simulink model "base_1fm"  (R2016b)
settings: Solver=VariableStepAuto  StartTime=0.0  StopTime=10.0  RelTol=1e-3
values from neighbouring files (symbols this model uses):
  Lb = 0.07    [base_1fm_parameters.m]
  Lf = 0.238    [base_1fm_parameters.m]
  Lu = 0.153    [base_1fm_parameters.m]
  sampleTime = 0.001    [base_1fm_parameters.m]
undefined symbols (not defined in the file or in its folder): DiscIntNeverNeededParam, RobotStruct
undefined symbols (not defined in the file): RobotStruct_FM1
libraries: simulink x27, VariousBlocksLibrary x4, FMLibrary_v2 x2, UsefulBlocksLibrary x2, simulink_extras x2, FM_Library x1
(part 3 of 3)

== matlab function base_1fm/Robot1/DataFromEtherCAT/FromActuator2/CalculateJointVelocity/FOAW ==
  data: x input; xdot output; sampleTime parameter; noise input
function xdot = foaw(x, sampleTime, noise)
%#codegen

SIZE = 100; % number of samples in buffer
NOISE = noise;
Ts = sampleTime;

persistent posbuffer;
persistent buffercntr;

% initialize buffer
if isempty(posbuffer)
    posbuffer = zeros(SIZE,1); % 1D case for now
    buffercntr = 0;
end

% fill buffer: shift data and add new value (loose oldest sample)
posbuffer = [posbuffer(2:end); x];
buffercntr = buffercntr + 1;
if buffercntr > SIZE, buffercntr = SIZE; end;

% if buffercntr = 1, only 1 data point is available, and you can't make a
% velocity prediction based on 1 data point. Set velocity ot 0, and return
% function
xdot = 0;
if buffercntr <= 3
    return;
end

for n = 1:buffercntr-1 % n = window size
        
    % step 2
    currentpos = posbuffer(end);

    % step 3 - calculate LS approximation of slope (hence velocity)
    b = n*sum(posbuffer(end-n:end)) - 2*sum(posbuffer(end-n:end).*(n:-1:0)');
    b = b / (Ts*n*(n+1)*(n+2)/6);

    % step 4 - check whether the line an + bn*Ts passes through all points inside the 
    % window within the uncertainty band of each point 
    jj = 0:n;
    yk_hat = currentpos-(b*jj*Ts);
    yk = posbuffer(end-jj)';
    if any(abs(yk_hat-yk) > NOISE)
        break;
    end

    xdot = b;
end

== matlab function base_1fm/Robot1/DataFromEtherCAT/FromActuator1/CalculateJointVelocity/FOAW ==
  data: x input; xdot output; sampleTime parameter; noise input
function xdot = foaw(x, sampleTime, noise)
%#codegen

SIZE = 100; % number of samples in buffer
NOISE = noise;
Ts = sampleTime;

persistent posbuffer;
persistent buffercntr;

% initialize buffer
if isempty(posbuffer)
    posbuffer = zeros(SIZE,1); % 1D case for now
    buffercntr = 0;
end

% fill buffer: shift data and add new value (loose oldest sample)
posbuffer = [posbuffer(2:end); x];
buffercntr = buffercntr + 1;
if buffercntr > SIZE, buffercntr = SIZE; end;

% if buffercntr = 1, only 1 data point is available, and you can't make a
% velocity prediction based on 1 data point. Set velocity ot 0, and return
% function
xdot = 0;
if buffercntr <= 3
    return;
end

for n = 1:buffercntr-1 % n = window size
        
    % step 2
    currentpos = posbuffer(end);

    % step 3 - calculate LS approximation of slope (hence velocity)
    b = n*sum(posbuffer(end-n:end)) - 2*sum(posbuffer(end-n:end).*(n:-1:0)');
    b = b / (Ts*n*(n+1)*(n+2)/6);

    % step 4 - check whether the line an + bn*Ts passes through all points inside the 
    % window within the uncertainty band of each point 
    jj = 0:n;
    yk_hat = currentpos-(b*jj*Ts);
    yk = posbuffer(end-jj)';
    if any(abs(yk_hat-yk) > NOISE)
        break;
    end

    xdot = b;
end

== matlab function base_1fm/Robot1/DataToEtherCAT/FTSensorError/MATLAB Function ==
  data: ForcesTorques input; e output; MaxForcesTorques input
function e = fcn(ForcesTorques, MaxForcesTorques)

% throw error when any of the forces/torques go over a max allowable value
if any(abs(ForcesTorques) > MaxForcesTorques) 
    e = 1;
else
    e = 0;
end

== matlab function base_1fm/Robot1/DataFromEtherCAT/FromActuator2/CalibrateAbsEncoder ==
  data: encoderPosition input; JointPosition_AbsEnc_rad output; offset input
function JointPosition_AbsEnc_rad = CalibrateAbsoluteEncoder(encoderPosition, offset)
%#codegen

% unwrap encoder angle (in case the encoder goes through 0
encoderPosition = unwrap(encoderPosition);

% remove offset
JointPosition_AbsEnc_rad = encoderPosition - offset;

% since the absolute encoder is mounted upside-down, negate the
% jointposition angle
JointPosition_AbsEnc_rad = -JointPosition_AbsEnc_rad;

== matlab function base_1fm/Robot1/DataFromEtherCAT/FromActuator2/CalibrateMotorPosition     ==
  data: JointPosition_IncEnc_rad output; MotorPosition_rad input; MotorPositionCalibrated_rad output; transmissionRatio parameter; JointPosition_AbsEnc_rad input; Calibrate input
function [JointPosition_IncEnc_rad,MotorPositionCalibrated_rad]...
    = CalibrateMotorPosition( MotorPosition_rad, transmissionRatio, JointPosition_AbsEnc_rad, Calibrate)
%#codegen

% This block includes calibration such that (ideally) the motor angle is
% zero when the joint angle and spring deflection are zero as well. Before
% the calibration has occurred, the output of this function is -1e9*. This
% is chosen such that the value is always outside the allowed motor angle
% range; this prevents the drive from being allowed to turn on.
% 
% * I wanted to use -inf as starting function, but I'm not sure whether
%   that will be handled correctly in all cases.

persistent isCalibrated;
persistent offset;

if isempty(isCalibrated) % no calibration needed
    isCalibrated = 1;
    offset = 0;
end;


if Calibrate
%     if ~isempty(JointPosition_AbsEnc_rad)
        target_pos_mot_rad = transmissionRatio * JointPosition_AbsEnc_rad; % This is what we should read
%         target_pos_mot_rad = CalibrationAngle; % This is what we should read / fix for now
        offset = target_pos_mot_rad - MotorPosition_rad; % calculate offset
%     else
%         % no absolute encoder data available, offset is zero
%         offset = 0;
%     end
    isCalibrated = 1;
end;

% if already calibrated, calculate calibrated motor angle
if isCalibrated
    MotorPositionCalibrated_rad = MotorPosition_rad + offset;
    JointPosition_IncEnc_rad = MotorPositionCalibrated_rad / transmissionRatio;
else
    MotorPositionCalibrated_rad = MotorPosition_rad;
    JointPosition_IncEnc_rad = MotorPositionCalibrated_rad / transmissionRatio;
end;

== matlab function base_1fm/Robot1/DataFromEtherCAT/FromActuator2/CheckOperationEnabled ==
  data: u input; y output
function y = fcn(u)
%#codegen

mask  = bin2dec('0000000001101111');
match = bin2dec('0000000000100111');

masked = bitand(u,mask);
if masked==match
    y=1;
else
    y=0;
end;

== matlab function base_1fm/Robot1/Controller/PD + Nonlinear ID/AFFC/AFFC ==
  data: p output; t input; q input; qdot input; qddot input; e input; tau output; Lf parameter; Lu parameter; Lb parameter; w input
function [p,tau] = fcn(t, q, qdot, qddot, e, Lf, Lu, Lb,w)

persistent p_;

if isempty(p_)
%     p_ = [0.00173;0.00159;0.048;0.07889;-0.00389;0.08784;-0.00474];
    p_ = zeros(7,1);
end


% jacobians
J = func_eq_Je(q(1),q(2),Lf,Lu,Lb);
Jdot = func_eq_Jedot(q(1),q(2),qdot(1),qdot(2),Lf,Lu,Lb);

% create Psi
Psi = [diag([qddot(1) qddot(2)]) J'*J*qddot+J'*Jdot*qdot [sign(qdot(1)) qdot(1); 0 0] [0 0;sign(qdot(2)) qdot(2)] ];

% learning matrix Gamma
eta = 0.95*exp(-t/150) + 0.05;
% eta = 1;
% wI = 1e-3;
% wme = 5e-2;
% wfd = 1e-3;
% wfs = 1e-3;

wI = w(1);
wme = w(2);
wfd = w(3);
wfs = w(4);

Gamma = eta*diag([wI wI wme wfs wfd wfs wfd]);

% update p (parameter vector)
% learning rule
dp = Gamma*Psi'*e;
p_ = p_ + dp;

% Psi = [diag([qddot(1) qddot(2)]) J'*J*qddot+J'*Jdot*qdot [ssign(qdot(1)) qdot(1); 0 0] [0 0;ssign(qdot(2)) qdot(2)] ];

% feedforward torque
tau = Psi*p_;

p = p_;

function y = ssign(u,beta)
% soft sign
if nargin == 1
    beta = 150;
end

y = 2./(1+exp(-beta*u))-1;

== stateflow chart base_1fm/Robot1/StateMachineLocal/SystemLocalStateMachine ==
  settings: initializeOutput=1
  state Operational
    state Calibration
      en:
      systemState = 2;
      velBelowThreshold = false;
      du:
      velBelowThreshold = checkVelThreshold(0.001 );
      state JointVelLarge
      state JointVelSmall
      state DoCalibration
        en: systemState = 201;
      state CalibrationDone
        en: systemState = 299;
      (default) -> JointVelLarge
      JointVelSmall -> JointVelLarge [order 1] : [!velBelowThreshold]
      JointVelLarge -> JointVelSmall : [velBelowThreshold]
      JointVelSmall -> DoCalibration [order 2] : after(2,sec)
      DoCalibration -> CalibrationDone
    state Homing
      en:
      systemState = reqSystemState;
      isAtHome = false;
      du:
      isAtHome = checkEndpointPosition(homeLocationSize);
      state NotAtHome
      state AtHome
      state HomingDone
        en: systemState = 399;
      (default) -> NotAtHome
      AtHome -> NotAtHome [order 1] : [!isAtHome]
      NotAtHome -> AtHome : [isAtHome]
      AtHome -> HomingDone [order 2] : after(1,sec)
    state Run
      en: systemState = 4;
    (default) -> Calibration
    CalibrationDone -> Homing : [reqSystemState == 301 || reqSystemState == 302]
    Run -> Homing : [reqSystemState==3]
    HomingDone -> Run : [reqSystemState==4]
  state Idle
    en:
    systemState = 0;
  state Init
    en:
    systemState = 1;
    du:
    isInitialized = true;
  state Error
    en: systemState=-1;
  (default) -> Idle
  Init -> Operational [order 1] : [isInitialized]
  Idle -> Init [order 2] : [reqSystemState==1]
  Init -> Idle [order 3] : [reqSystemState==0]
  Error -> Idle : [!error   && reqSystemState==0]
  Init -> Error [order 2] : [error]
  Idle -> Error [order 1] : [error]
  Operational -> Idle [order 2] : [reqSystemState==0]
  Operational -> Error [order 1] : [error]
  data: threshold function_input double; velIsUnderThreshold function_output boolean; threshold function_input double; isAtEndpoint function_output boolean; reqSystemState input double; currentSystemState output double; error input boolean; x input double; xdot input double; HomePosition input double; isAtHome local boolean; velBelowThreshold local boolean; isInitialized local double; homeLocationSize input
  function velIsUnderThreshold = checkVelThreshold(threshold):
    | function velIsUnderThreshold = checkVelThreshold(threshold)
    |  
    | velIsUnderThreshold = all(abs(xdot) <= threshold);
  function isAtEndpoint = checkEndpointPosition(threshold):
    | function isAtEndpoint = checkEndpointPosition(threshold)
    | % check whether the endpoint position is within a specified circle with
    | % radius threshold and midopoint HomePosition
    | 
    | % calculate distance between home position and joint positions
    | d = sqrt(sum((HomePosition - x).^2));
    | 
    | if imag(d) || isinf(d) || isnan(d)
    |     isAtEndpoint = false;
    | else
    |     isAtEndpoint = d <= threshold;
    | end

== matlab function base_1fm/Robot1/StateMachineLocal/Encode system state change ==
  data: stateChanged input; state input; systemStateChanged output
function systemStateChanged  = fcn(stateChanged,state)

systemStateChanged = 0;


if stateChanged
    switch(state)
        case 201 % do calibration
            systemStateChanged = 1;
    end
end

== matlab function base_1fm/Robot1/DataFromEtherCAT/Calculate Arrange Joint and Op Space/forward kinematics/forward kinematics ==
  data: q input; x output size=[2 1]; Lf parameter; Lu parameter; Lb parameter
function x = FK(q, Lf, Lu, Lb)
%#codegen

% Calculate the endpoint position (forward kinematics)
% Note that the function func_eq_FK needs to be in the libraries/kinematis_functions folder


x = func_eq_FK(q(1),q(2),Lf,Lu,Lb);

== matlab function base_1fm/Robot1/DataFromEtherCAT/FromActuator2/DecodeActualTorque ==
  data: JointTorque_Act_Nm output; MotorCurrent_Act_IU input int16; transmissionRatio parameter; drivePeakCurrent parameter; motorTorqueConstant parameter
function JointTorque_Act_Nm = DecodeActualTorque(MotorCurrent_Act_IU, transmissionRatio, drivePeakCurrent, motorTorqueConstant)
%#codegen
%

% convert incremental units to motor torque value. See the technosoft CoE
% manual for the decoding
torquemotor_act = motorTorqueConstant * (double(MotorCurrent_Act_IU)*2*drivePeakCurrent / 65520);

% motor torque to joint torque (transmission). Negate due to sign change
% due to transmission.
JointTorque_Act_Nm = torquemotor_act * transmissionRatio;

== matlab function base_1fm/Robot1/DataFromEtherCAT/FromActuator2/DecodeEncoder_AbsEnc ==
  data: Encoder_counts input; EncoderCounts_rev parameter; EncoderPosition_rad output
function EncoderPosition_rad = ...
    DecodeEncoder(Encoder_counts, EncoderCounts_rev)
%#codegen

% This block decodes the motor encoder counts to the motor angle

EncoderPosition_rad = (double(Encoder_counts) / EncoderCounts_rev * 2 * pi);

== matlab function base_1fm/Robot1/Controller/inverse kinematics1 ==
  data: x input; q output size=[2 1]; Lf parameter; Lu parameter; Lb parameter
function q  = IK(x,Lf,Lu,Lb)
%#codegen

% inverse dynamics
q = func_eq_IK(x(1),x(2),Lf,Lu,Lb);

== matlab function base_1fm/Robot1/DataFromEtherCAT/FromActuator2/DecodeEncoder_IncEnc ==
  data: Encoder_counts input; EncoderCounts_rev parameter; EncoderPosition_rad output
function EncoderPosition_rad = ...
    DecodeEncoder(Encoder_counts, EncoderCounts_rev)
%#codegen

% This block decodes the motor encoder counts to the motor angle

EncoderPosition_rad = (double(Encoder_counts) / EncoderCounts_rev * 2 * pi);

== matlab function base_1fm/Robot1/DataFromEtherCAT/FromActuator1/CalibrateMotorPosition     ==
  data: JointPosition_IncEnc_rad output; MotorPosition_rad input; MotorPositionCalibrated_rad output; transmissionRatio parameter; JointPosition_AbsEnc_rad input; Calibrate input
function [JointPosition_IncEnc_rad,MotorPositionCalibrated_rad]...
    = CalibrateMotorPosition( MotorPosition_rad, transmissionRatio, JointPosition_AbsEnc_rad, Calibrate)
%#codegen

% This block includes calibration such that (ideally) the motor angle is
% zero when the joint angle and spring deflection are zero as well. Before
% the calibration has occurred, the output of this function is -1e9*. This
% is chosen such that the value is always outside the allowed motor angle
% range; this prevents the drive from being allowed to turn on.
% 
% * I wanted to use -inf as starting function, but I'm not sure whether
%   that will be handled correctly in all cases.

persistent isCalibrated;
persistent offset;

if isempty(isCalibrated) % no calibration needed
    isCalibrated = 1;
    offset = 0;
end;


if Calibrate
%     if ~isempty(JointPosition_AbsEnc_rad)
        target_pos_mot_rad = transmissionRatio * JointPosition_AbsEnc_rad; % This is what we should read
%         target_pos_mot_rad = CalibrationAngle; % This is what we should read / fix for now
        offset = target_pos_mot_rad - MotorPosition_rad; % calculate offset
%     else
%         % no absolute encoder data available, offset is zero
%         offset = 0;
%     end
    isCalibrated = 1;
end;

% if already calibrated, calculate calibrated motor angle
if isCalibrated
    MotorPositionCalibrated_rad = MotorPosition_rad + offset;
    JointPosition_IncEnc_rad = MotorPositionCalibrated_rad / transmissionRatio;
else
    MotorPositionCalibrated_rad = MotorPosition_rad;
    JointPosition_IncEnc_rad = MotorPositionCalibrated_rad / transmissionRatio;
end;

== matlab function base_1fm/Robot1/Controller/homing - active/Filter1 ==
  data: x input; OmegaFilter input; y output; sampleTime parameter
function y = Filter2ndOrder(x, OmegaFilter, sampleTime)
%#codegen

persistent yd_prev y_prev;
if isempty(yd_prev)
    yd_prev = 0; 
    y_prev = 0; %Derivative of the above signal
end;

% Do 2nd order filtering with given omega and zeta=0.7; input of filter
% is vel_inc_sampleTime_unfilt; output is y (we assign to vel_inc_s
% later). 
if OmegaFilter==0 || isinf(OmegaFilter)
    y=x;
    y_prev=y;
    yd_prev =0;
else
    zeta = 0.7;
    ydd = OmegaFilter^2 * (x - y_prev) - 2*zeta*OmegaFilter* yd_prev;
    yd = yd_prev + ydd * sampleTime;
    y = y_prev + yd * sampleTime;

    y_prev = y; yd_prev = yd;
end;

== matlab function base_1fm/Haptics/Hypotrochoid trajectory for AFFC/hypotrochoidal trajectory ==
  data: t input; p output; v output; a output; T input; n input; hstart input; hend input; wstart input; wend input
function [p,v,a] = fcn(t,T,n,hstart,hend,wstart,wend)
%#codegen

p = func_p_hypothrochoid(t,T,n,hstart,hend,wstart,wend);
v = func_v_hypothrochoid(t,T,n,hstart,hend,wstart,wend);
a = func_a_hypothrochoid(t,T,n,hstart,hend,wstart,wend);

== matlab function base_1fm/Robot1/DataToEtherCAT/ToActuator1/DriveEnableLogic/64_DriveError/CountHowLongEnableWasTrue ==
  data: u input; y output
function y = fcn(u)
%#codegen
%
% This block counts how many samples the input has been on (true). As soon
% as the input goes false, the counter is reset.
persistent onCounter;

if isempty(onCounter)
    onCounter = 0;
end;

if u == 1
    onCounter = onCounter + 1;
else
    % u == 0
    onCounter = 0;
end;
y = onCounter;

== matlab function base_1fm/Robot1/DataFromEtherCAT/Calculate Arrange Joint and Op Space/forward kinematics/Je ==
  data: q input; Je output size=[2 2]; Lf parameter; Lu parameter; Lb parameter
function Je = Je( q, Lf, Lu, Lb)
%#codegen

% Calculate the Jacobian for this particular device configuration.
% Note that the function func_eq_Je needs to be in the libraries/kinematis_functions folder

% jacobians
Je = func_eq_Je(q(1),q(2),Lf,Lu,Lb);

== matlab function base_1fm/Robot1/DataFromEtherCAT/Calculate Arrange Joint and Op Space/forward kinematics/Jedot ==
  data: q input; qdot input; Jedot output size=[2 2]; Lf parameter; Lu parameter; Lb parameter
function Jedot = Jedot( q, qdot, Lf, Lu, Lb)
%#codegen

% Calculate the time derivative of the Jacobian for this particular device configuration.
% Note that the function func_eq_Je needs to be in the libraries/kinematis_functions folder


% jacobians
Jedot = func_eq_Jedot(q(1),q(2),qdot(1),qdot(2),Lf,Lu,Lb);

== matlab function base_1fm/Robot1/DataFromEtherCAT/FTSensor_K6D27/CorrectOffset ==
  data: u_in input; u_out output; reset input; corrected output
function [u_out,corrected] = CorrectOffset(u_in,reset)
%#codegen

persistent data_ offset_ counter_ corrected_;
N = 1000;

% initialize
if isempty(data_)
    data_ = zeros(size(u_in,1), N);
    offset_ = zeros(size(u_in));
    counter_ = 1;
    corrected_ = 0;
end

if (counter_ <= N)
    data_(:,counter_) = u_in;
end

counter_ = counter_ + 1;
if reset
    counter_ = 1;
end

% calculate mean
if counter_ == N
    corrected_ = 1;
    offset_ = mean(data_,2);
end

corrected = corrected_;
u_out = u_in - offset_;

== matlab function base_1fm/Robot1/DataFromEtherCAT/FromActuator1/CheckOperationEnabled ==
  data: u input; y output
function y = fcn(u)
%#codegen

mask  = bin2dec('0000000001101111');
match = bin2dec('0000000000100111');

masked = bitand(u,mask);
if masked==match
    y=1;
else
    y=0;
end;

== matlab function base_1fm/Robot1/DataFromEtherCAT/Calculate Arrange Joint and Op Space/IK all joints ==
  data: x input; q_all output; Lf parameter; Lu parameter; Lb parameter
function q_all = IK_all(x,Lf,Lu,Lb)
%#codegen

if (x(2) >= 0.07)
    q_all = func_eqs_IK_all(x(1),x(2),Lf,Lu,Lb);
else
    x = [0;0.07];
    q_all = func_eqs_IK_all(x(1),x(2),Lf,Lu,Lb);
end

== matlab function base_1fm/Robot1/DataFromEtherCAT/Calculate Arrange Joint and Op Space/forward kinematics/calculate xddot ==
  data: qddot input; qdot input size=[2 1]; J input; xddot output size=[2 1]; Jdot input
function xddot = calc_xddot(qddot, qdot, J, Jdot)
%#codegen

xddot = J*qddot + Jdot*qdot;

== matlab function base_1fm/Robot1/Controller/inverse kinematics ==
  data: x input; xdot input; xddot input; q output size=[2 1]; Lf parameter; Lu parameter; Lb parameter; qdot output; qddot output
function [q,qdot,qddot] = IK(x,xdot,xddot,Lf,Lu,Lb)
%#codegen

% inverse dynamics
q = func_eq_IK(x(1),x(2),Lf,Lu,Lb);

% jacobians
Je = func_eq_Je(q(1),q(2),Lf,Lu,Lb);

% calculate qdot
qdot = pinv(Je)*xdot;

% calculate qddot
Jedot = func_eq_Jedot(q(1),q(2),qdot(1),qdot(2),Lf,Lu,Lb);
qddot = pinv(Je)*(xddot-Jedot*qdot);

== matlab function base_1fm/Robot1/DataToEtherCAT/ToActuator1/DriveEnableLogic/CreateSingleErrorValue/MATLAB Function ==
  data: errors input; out output
function out = errorToPowerOf2(errors)
%#codegen

% if size(errors,1) > size(errors,2)
%     errors = errors.';
% end
out = sum(errors.*(2.^(0:(length(errors)-1)).'));

== matlab function base_1fm/Robot1/DataToEtherCAT/ToActuator1/DriveEnableLogic/enableDrive (CoE) ==
  data: ControlWord output; enable input; TimePerState_ms input
function ControlWord = enabledrive(enable, TimePerState_ms)
%#codegen
%
% Input arguments:
% enable:
%   0: Disable drive
%   Any non-zero: enable drive.
% TimePerState_ms:
%   A four-element array containing the time in ms for each state (states
%   are: 0, 128, 6, 7. The final state, 15, is kept until drive needs to be
%   disabled again.
%
% Changing enable forces the initialize-sequence to run
persistent previousEnable;
persistent counter;
if isempty(previousEnable)
    previousEnable = enable; % No enabling of the drive at startup
    counter = 1e6;
end;

if enable~=previousEnable
    counter = 0;
end;
previousEnable = enable;

TimePerState_cum = cumsum(TimePerState_ms);

if enable~=0
    counter = counter+1;
    if counter < TimePerState_cum(1);
        ControlWord_ = 0;
    elseif counter < TimePerState_cum(2);
        ControlWord_ = 128;
    elseif counter < TimePerState_cum(3);
        ControlWord_ = 6;
    elseif counter < TimePerState_cum(4);
        ControlWord_ = 7;
    else
        ControlWord_ = 15;
    end
else
    ControlWord_ = 6;
end

ControlWord = uint16(ControlWord_);

== matlab function base_1fm/Robot1/DataToEtherCAT/ToActuator1/EncodeDesiredTorque ==
  data: MotorTorque_Des_IU output int16; JointTorque_Des_Nm input; transmissionRatio parameter; motorTorqueConstant parameter; drivePeakCurrent parameter
function MotorTorque_Des_IU = EncodeDesiredTorque(JointTorque_Des_Nm, transmissionRatio, motorTorqueConstant, drivePeakCurrent)
%#codegen
% Calculate the target torque in incremental units for a desired joint
% torque.

% compute torque at motor (negate because sign change due to transmission)
torque_motor = JointTorque_Des_Nm / transmissionRatio; 

% desired current (i_des) = torque_motor / kt (torque constant)
i_des = torque_motor / motorTorqueConstant;

% calculate the target torque in incremental units [IU], see CoE manual
% Technosoftmotion
MotorTorque_Des_IU = int16( 65520*i_des / (2*drivePeakCurrent) );

== matlab function base_1fm/Robot1/DataToEtherCAT/ToActuator/DriveEnableLogic/64_DriveError/CountHowLongEnableWasTrue ==
  data: u input; y output
function y = fcn(u)
%#codegen
%
% This block counts how many samples the input has been on (true). As soon
% as the input goes false, the counter is reset.
persistent onCounter;

if isempty(onCounter)
    onCounter = 0;
end;

if u == 1
    onCounter = onCounter + 1;
else
    % u == 0
    onCounter = 0;
end;
y = onCounter;

== matlab function base_1fm/Robot1/DataFromEtherCAT/FromActuator1/DecodeActualTorque ==
  data: JointTorque_Act_Nm output; MotorCurrent_Act_IU input int16; transmissionRatio parameter; drivePeakCurrent parameter; motorTorqueConstant parameter
function JointTorque_Act_Nm = DecodeActualTorque(MotorCurrent_Act_IU, transmissionRatio, drivePeakCurrent, motorTorqueConstant)
%#codegen
%

% convert incremental units to motor torque value. See the technosoft CoE
% manual for the decoding
torquemotor_act = motorTorqueConstant * (double(MotorCurrent_Act_IU)*2*drivePeakCurrent / 65520);

% motor torque to joint torque (transmission). Negate due to sign change
% due to transmission.
JointTorque_Act_Nm = torquemotor_act * transmissionRatio;

== matlab function base_1fm/Robot1/DataFromEtherCAT/FromActuator1/DecodeEncoder_AbsEnc ==
  data: Encoder_counts input; EncoderCounts_rev parameter; EncoderPosition_rad output
function EncoderPosition_rad = ...
    DecodeEncoder(Encoder_counts, EncoderCounts_rev)
%#codegen

% This block decodes the motor encoder counts to the motor angle

EncoderPosition_rad = (double(Encoder_counts) / EncoderCounts_rev * 2 * pi);

== matlab function base_1fm/Robot1/DataFromEtherCAT/FromActuator1/DecodeEncoder_IncEnc ==
  data: Encoder_counts input; EncoderCounts_rev parameter; EncoderPosition_rad output
function EncoderPosition_rad = ...
    DecodeEncoder(Encoder_counts, EncoderCounts_rev)
%#codegen

% This block decodes the motor encoder counts to the motor angle

EncoderPosition_rad = (double(Encoder_counts) / EncoderCounts_rev * 2 * pi);

== matlab function base_1fm/Robot1/DataFromEtherCAT/FromActuator1/CalibrateAbsEncoder ==
  data: encoderPosition input; JointPosition_AbsEnc_rad output; offset input
function JointPosition_AbsEnc_rad = CalibrateAbsoluteEncoder(encoderPosition, offset)
%#codegen

% unwrap encoder angle (in case the encoder goes through 0
encoderPosition = unwrap(encoderPosition);

% remove offset
JointPosition_AbsEnc_rad = encoderPosition - offset;

% since the absolute encoder is mounted upside-down, negate the
% jointposition angle
JointPosition_AbsEnc_rad = -JointPosition_AbsEnc_rad;

== matlab function base_1fm/Robot1/DataToEtherCAT/ToActuator/DriveEnableLogic/CreateSingleErrorValue/MATLAB Function ==
  data: errors input; out output
function out = errorToPowerOf2(errors)
%#codegen

% if size(errors,1) > size(errors,2)
%     errors = errors.';
% end
out = sum(errors.*(2.^(0:(length(errors)-1)).'));

== matlab function base_1fm/Robot1/DataToEtherCAT/ToActuator/DriveEnableLogic/enableDrive (CoE) ==
  data: ControlWord output; enable input; TimePerState_ms input
function ControlWord = enabledrive(enable, TimePerState_ms)
%#codegen
%
% Input arguments:
% enable:
%   0: Disable drive
%   Any non-zero: enable drive.
% TimePerState_ms:
%   A four-element array containing the time in ms for each state (states
%   are: 0, 128, 6, 7. The final state, 15, is kept until drive needs to be
%   disabled again.
%
% Changing enable forces the initialize-sequence to run
persistent previousEnable;
persistent counter;
if isempty(previousEnable)
    previousEnable = enable; % No enabling of the drive at startup
    counter = 1e6;
end;

if enable~=previousEnable
    counter = 0;
end;
previousEnable = enable;

TimePerState_cum = cumsum(TimePerState_ms);

if enable~=0
    counter = counter+1;
    if counter < TimePerState_cum(1);
        ControlWord_ = 0;
    elseif counter < TimePerState_cum(2);
        ControlWord_ = 128;
    elseif counter < TimePerState_cum(3);
        ControlWord_ = 6;
    elseif counter < TimePerState_cum(4);
        ControlWord_ = 7;
    else
        ControlWord_ = 15;
    end
else
    ControlWord_ = 6;
end

ControlWord = uint16(ControlWord_);

== matlab function base_1fm/Robot1/DataToEtherCAT/ToActuator/EncodeDesiredTorque ==
  data: MotorTorque_Des_IU output int16; JointTorque_Des_Nm input; transmissionRatio parameter; motorTorqueConstant parameter; drivePeakCurrent parameter
function MotorTorque_Des_IU = EncodeDesiredTorque(JointTorque_Des_Nm, transmissionRatio, motorTorqueConstant, drivePeakCurrent)
%#codegen
% Calculate the target torque in incremental units for a desired joint
% torque.

% compute torque at motor (negate because sign change due to transmission)
torque_motor = JointTorque_Des_Nm / transmissionRatio; 

% desired current (i_des) = torque_motor / kt (torque constant)
i_des = torque_motor / motorTorqueConstant;

% calculate the target torque in incremental units [IU], see CoE manual
% Technosoftmotion
MotorTorque_Des_IU = int16( 65520*i_des / (2*drivePeakCurrent) );

== matlab function base_1fm/Robot1/DataFromEtherCAT/FTSensor_K6D27/SensorOutputToForce1 ==
  data: FT output; u input; calibrationMatrix input; offset input
function FT = VtoF(u, calibrationMatrix, offset)
%#codegen

% ME supplies a zero offset voltages. If 
if ~isempty(offset)
    u = u + offset;
end

% Calculate forces and torques (in sensor space)
FT = calibrationMatrix*u;

== matlab function base_1fm/Robot1/DataFromEtherCAT/FTSensor_K6D27/SensorToOperationalSpace ==
  data: q_all input; Fs input; FTOpSpace output
function FTOpSpace = ForceSensorToOperationalSpace(q_all,Fs)
%#codegen

% select correct angles. Note! During assembly we weren't very consistent
% to which forearm the sensor is fixed. For FM1 (green), the sensor is
% attached to arm 2, hence the rotation matrics are made using angles
% theta1 and theta2
% rotation matrices (I derived them from actuator 1 to endpoint, but
% transformation is other way around (i.e. inverse). Since inverse calculation 
% could take some time, Could be done by
% negating the angles instead of inverse of matrix.
q1 = q_all(1);
q2 = (pi-q_all(2)); % pi-theta2 since theta2 is the internal angle of this joint

R = [-cos(q1+q2) sin(q1+q2);-sin(q1+q2) -cos(q1+q2)];

% transform force
FTOpSpace = R*Fs(1:2);

== matlab function base_1fm/Robot1/DataToEtherCAT/WorkspacePositionGuard/CheckForSingularity ==
  data: J input; kappa output
function kappa = conditionnumber(J)
%#codegen

kappa = norm(pinv(J))*norm(J);

== matlab function base_1fm/Robot1/DataToEtherCAT/WorkspacePositionGuard/CheckInternalAngles ==
  data: theta input; angleError output; isCalibrated input
function angleError = checkInternalErrors(theta,isCalibrated)
%#codegen

angleError = 0;

if isCalibrated
    % check whether theta2 or theta4 are smaller than 0.95*pi. If larger, throw
    % error
    if any(theta([2 4]) >= 0.95*pi)
        angleError = 1;
    end
end

== matlab function base_1fm/Robot1/DataToEtherCAT/WorkspacePositionGuard/CreateSingleErrorValue/MATLAB Function ==
  data: errors input; out output
function out = errorToPowerOf2(errors)
%#codegen

% if size(errors,1) > size(errors,2)
%     errors = errors.';
% end
out = sum(errors.*(2.^(0:(length(errors)-1)).'));

== matlab function base_1fm/Robot1/DataToEtherCAT/WorkspacePositionGuard/EndpointPositionGuard ==
  data: xe input; error output; correctState input
function error = fcn(xe, correctState)
%#codegen


error = 0;

% only check workspace boundaries after homing state is done
if ~correctState 
    return; 
end

% x0 = 0;
% y0 = 0.2354;
% a = 0.11;
% b = 0.08;

% workspace (see design document)
x0 = 0;
y0 = 0.25024;
a = 0.1746;
b = 0.13;%0.1048;

% check if endpoint is outside a predefined ellipse
x = xe(1);
y = xe(2);

% workspace is defined as an ellipse
e = (x-x0)^2 / a^2 + (y-y0)^2 / b^2;

% if is larger than 1, the endpoint is outside the workspace
if e > 1
    error = 1;
end
